simulink model "CrCtl_StM"  (R2016b)
settings: configuration reference "CodeGenConfigSet" (kept outside this file)
values from neighbouring files (symbols this model uses):
  CrCtl_aAccThres_C = Calibration.Parameter    [init_CrCtl_StM.m]
  CrCtl_aDeclThres_C = Calibration.Parameter    [init_CrCtl_StM.m]
  CrCtl_facRmpSlpAcc_C = Calibration.Parameter    [init_CrCtl_StM.m]
  CrCtl_facRmpSlpDecl_C = Calibration.Parameter    [init_CrCtl_StM.m]
  CrCtl_facRmpSlpRes_C = Calibration.Parameter    [init_CrCtl_StM.m]
  CrCtl_swtOffTipDwnTrqLim_C = Calibration.Parameter    [init_CrCtl_StM.m]
  CrCtl_swtOffTipUpTrqLim_C = Calibration.Parameter    [init_CrCtl_StM.m]
  CrCtl_trqLimOffsetAcc_C = Calibration.Parameter    [init_CrCtl_StM.m]
  CrCtl_trqLimOffsetDecl_C = Calibration.Parameter    [init_CrCtl_StM.m]
  CrCtl_vDvtMaxAccDecl_C = Calibration.Parameter    [init_CrCtl_StM.m]
  CrCtl_vMaxDvtAcc_C = Calibration.Parameter    [init_CrCtl_StM.m]
  CrCtl_vMaxDvtDecl_C = Calibration.Parameter    [init_CrCtl_StM.m]
  CrCtl_vMaxDvtResAbv_C = Calibration.Parameter    [init_CrCtl_StM.m]
  CrCtl_vMaxDvtResBlw_C = Calibration.Parameter    [init_CrCtl_StM.m]
  CrCtl_vTipDwnDvtn_C = Calibration.Parameter    [init_CrCtl_StM.m]
  CrCtl_vTipDwnLoLim_C = Calibration.Parameter    [init_CrCtl_StM.m]
  CrCtl_vTipDwnUpLim_C = Calibration.Parameter    [init_CrCtl_StM.m]
  CrCtl_vTipStp_C = Calibration.Parameter    [init_CrCtl_StM.m]
  CrCtl_vTipUpDvtn_C = Calibration.Parameter    [init_CrCtl_StM.m]
  CrCtl_vTipUpLoLim_C = Calibration.Parameter    [init_CrCtl_StM.m]
  CrCtl_vTipUpUpLim_C = Calibration.Parameter    [init_CrCtl_StM.m]
  MoFDrAs_vCCtlMinCalMsg_C = Calibration.Parameter    [init_CrCtl_StM.m]
  VEL_ZERO = fi(0,VehSpeed_km_h)    [init_CrCtl_StM.m]
undefined symbols (not defined in the file or in its folder): CrCtl_stLck_conv, CrCtl_StM_DT, CrCtl_stShOff_conv, CrCtl_stSub_conv, CruiseCtl_State_conv
libraries: CXLib x15
(part 1 of 2)
settings Model: Creator=guanxiaoxing  LastModifiedBy=guanxiaoxing
settings ConfigSetRef: SourceLocation=Base Workspace

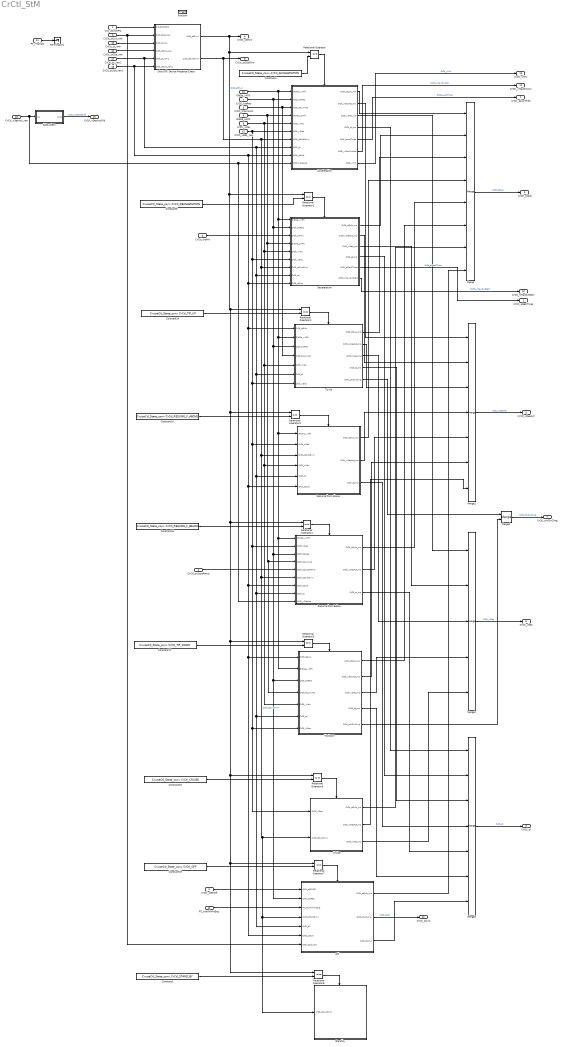
== system CrCtl_StM ==
  CrC_bCrCtlPrs : Inport  Description=Cruise control present status  OutMin=0  OutMax=1  OutDataTypeStr=boolean
  CrCtl_stLck_raw : Inport  Description=Cruise Control lock Status  Port=2  OutDataTypeStr=Enum: CrCtl_stLck_conv
  CrCtl_stShOff : Inport  Description=cruise control shut-off requirement  Port=3  OutDataTypeStr=Enum: CrCtl_stShOff_conv
  CrCtl_stSuspRamp : Inport  Description=Suspend ramp status  Port=4  OutDataTypeStr=Enum: CrCtl_stSuspRamp_conv
  CrCtl_trqLimAct : Inport  Tag=Nm  Description=Limited Cruise control torque  Port=5  OutMin=-3000  OutMax=3000  OutDataTypeStr=Trq_Nm
  CrCtl_trqMin : Inport  Tag=Nm  Description=cruise control desired torque when cruise control is inactive  Port=6  OutMin=-3000  OutMax=3000  OutDataTypeStr=Trq_Nm
  CrCtl_trqReq : Inport  Tag=Nm  Description=Cruise control torque request  Port=7  OutMin=-3000  OutMax=3000  OutDataTypeStr=Trq_Nm
  CrCtl_vMax : Inport  Tag=km/h  Description=Maximum speed for cruise control  Port=8  OutMin=0  OutMax=250  OutDataTypeStr=VehSpeed_km_h
  GlbDa_aXFlt : Inport  Tag=m/s^2  Description=Vehicle longitudinal acceleration filtered  Port=9  OutMin=-32  OutMax=32  OutDataTypeStr=Acc_m_s2
  GlbDa_vXFlt : Inport  Tag=km/h  Description=Vehicle velocity filtered  Port=10  OutMin=0  OutMax=250  OutDataTypeStr=VehSpeed_km_h
  PT_rTraV2N : Inport  Tag=km/h/rpm  Description=Quotient of velocity and engine speed  Port=11  OutMin=-0.32768  OutMax=0.32767  OutDataTypeStr=Tra_V2N_km_h_rpm
  PT_trqWhlMinEng : Inport  Tag=Nm  Description=Minimum wheel torque from the engine  Port=12  OutMin=-3000  OutMax=3000  OutDataTypeStr=Trq_Nm
  CrCtl_st_raw : Inport  Description=Application parameter for Cruise Control state  Port=13  OutDataTypeStr=Enum: CruiseCtl_State_conv
  CrCtl_stSub_raw : Inport  Description=Cruise control sub mode  Port=14  OutDataTypeStr=Enum: CrCtl_stSub_conv
  CrCtl_vDes_raw : Inport  Tag=km/h  Description=Cruise Control desired set point speed  Port=15  OutMin=0  OutMax=250  OutDataTypeStr=VehSpeed_km_h
  CrCtl_vDesAct_raw : Inport  Tag=km/h  Description=Target speed for cruise control  Port=16  OutMin=0  OutMax=250  OutDataTypeStr=VehSpeed_km_h
  CrCtl_st_raw1 : Inport  Description=Application parameter for Cruise Control state  Port=17  OutDataTypeStr=Enum: CruiseCtl_State_conv
  CrCtl_stSub_raw1 : Inport  Description=Cruise control sub mode  Port=18  OutDataTypeStr=Enum: CrCtl_stSub_conv
  function : TriggerPort  TriggerType=function-call  VariantControl=Variant
  Acceleration : Subsystem
  Constant1 : Constant  Value=CruiseCtl_State_conv.CrCtl_STAND_BY
  Constant14 : Constant  Value=CruiseCtl_State_conv.CrCtl_TIP_UP
  Constant15 : Constant  Value=CruiseCtl_State_conv.CrCtl_RESUME_F_ABOVE
  Constant16 : Constant  Value=CruiseCtl_State_conv.CrCtl_RESUME_F_BELOW
  Constant17 : Constant  Value=CruiseCtl_State_conv.CrCtl_TIP_DOWN
  Constant18 : Constant  Value=CruiseCtl_State_conv.CrCtl_CRUISE
  Constant19 : Constant  Value=CruiseCtl_State_conv.CrCtl_OFF
  Constant4 : Constant  Value=CruiseCtl_State_conv.CrCtl_ACCELERATION
  Constant6 : Constant  Value=CruiseCtl_State_conv.CrCtl_DECELERATION
  Cruise : Subsystem
  Deceleration : Subsystem
  Merge : Merge  Inputs=8
  Merge1 : Merge  Inputs=7
  Merge2 : Merge  Inputs=5
  Merge3 : Merge  Inputs=7
  Merge4 : Merge
  Off : Subsystem
  Relational Operator{,1..8} (9 alike) : RelationalOperator  Operator===  OutDataTypeStr=boolean  RndMeth=Simplest
  Resume from Above : Subsystem
  Resume from Below : Subsystem
  Shut Off / Device Presence Check : Subsystem
  Stand by : Subsystem
  Subsystem : Subsystem
  Terminator1 : Terminator
  Tip Down : Subsystem
  Tip Up : Subsystem
  CrCtl_aAccThres : Outport  Tag=m/s^2  Description=Accelration threshold for Cruise control  OutMin=-32  OutMax=32  OutDataTypeStr=Acc_m_s2
  CrCtl_aDeclThres : Outport  Tag=m/s^2  Description=Deaccelration threshold for Cruise control  Port=2  OutMin=-32  OutMax=32  OutDataTypeStr=Acc_m_s2
  CrCtl_st : Outport  Description=Application parameter for Cruise Control state  Port=3  OutDataTypeStr=Enum: CruiseCtl_State_conv
  CrCtl_stGvnr : Outport  Description=Governor status for cruise control  Port=4  OutDataTypeStr=Enum: CruiseCtl_State_conv
  CrCtl_stSub : Outport  Description=Cruise control sub mode  Port=5  OutDataTypeStr=Enum: CrCtl_stSub_conv
  CrCtl_stSubGvnr : Outport  Description=Cruise control sub mode for governor  Port=6  OutDataTypeStr=Enum: CrCtl_stSub_conv
  CrCtl_stVDirChng : Outport  Description=|  Port=7  OutMin=0  OutMax=1  OutDataTypeStr=boolean
      | Flag indicating if vehicle was under increasing speed request before and now speed decrease has
      | been request (or vice-versa)
  CrCtl_vDes : Outport  Tag=km/h  Description=Cruise Control desired set point speed  Port=8  OutMin=0  OutMax=250  OutDataTypeStr=VehSpeed_km_h
  CrCtl_vDesAct : Outport  Tag=km/h  Description=Target speed for cruise control  Port=9  OutMin=0  OutMax=250  OutDataTypeStr=VehSpeed_km_h
  CrCtl_vDesActOld : Outport  Tag=km/h  Description=Cruise control old active speed  Port=10  OutMin=0  OutMax=250  OutDataTypeStr=VehSpeed_km_h
  CrCtl_vMaxDvtAcc : Outport  Tag=km/h  Description=Maximum deviation speed for acceleration  Port=11  OutMin=0  OutMax=250  OutDataTypeStr=VehSpeed_km_h
  CrCtl_vMaxDvtDecl : Outport  Tag=km/h  Description=Maximum deviation speed for deacceleration  Port=12  OutMin=0  OutMax=250  OutDataTypeStr=VehSpeed_km_h
  CrCtl_vMin : Outport  Tag=km/h  Description=Minimum spped for cruise control  Port=13  OutMin=0  OutMax=250  OutDataTypeStr=VehSpeed_km_h
  CrCtl_stLck : Outport  Description=Cruise Control lock Status  Port=14  OutDataTypeStr=Enum: CrCtl_stLck_conv
  wires:
  Acceleration/5(CrCtl_aAccThres) -> CrCtl_aAccThres/1  "CrCtl_aAccThres"
  Deceleration/5(CrCtl_aDeclThres) -> CrCtl_aDeclThres/1  "CrCtl_aDeclThres"
  Merge3/1 -> CrCtl_st/1  "CrCtl_st"
  Shut Off / Device Presence Check/1(CrCtl_stGvnr) -> Relational Operator4/1, Relational Operator5/1, Relational Operator6/1, Relational Operator8/1, Relational Operator7/1, Relational Operator3/1, Relational Operator2/1, Relational Operator1/1, Relational Operator/1, CrCtl_stGvnr/1  "CrCtl_stGvnr"
  Merge/1 -> CrCtl_stSub/1  "CrCtl_stSub"
  Shut Off / Device Presence Check/2("CrCtl_stSubGvnr ") -> CrCtl_stSubGvnr/1, Resume from Below/6(CrCtl_stSubGvnr), Stand by/1(CrCtl_stSubGvnr), Off/4(CrCtl_stSubGvnr), Cruise/2(CrCtl_stSubGvnr), Resume from Above/3(CrCtl_stSubGvnr), Deceleration/7(CrCtl_stSubGvnr), Acceleration/7(CrCtl_stSubGvnr)  "CrCtl_stSubGvnr"
  Merge4/1 -> CrCtl_stVDirChng/1  "CrCtl_stVDirChng"
  Merge2/1 -> CrCtl_vDes/1  "CrCtl_vDes"
  Merge1/1 -> CrCtl_vDesAct/1  "CrCtl_vDesAct"
  Acceleration/6(" CrCtl_vMaxDvtAcc") -> CrCtl_vMaxDvtAcc/1  "CrCtl_vMaxDvtAcc"
  Deceleration/6(" CrCtl_vMaxDvtDecl") -> CrCtl_vMaxDvtDecl/1  "CrCtl_vMaxDvtDecl"
  Acceleration/7(" CrCtl_vMin") -> CrCtl_vMin/1  "CrCtl_vMin"
  PT_rTraV2N/1 -> Terminator1/1
  CrC_bCrCtlPrs/1 -> Shut Off / Device Presence Check/1(CrC_bCrCtlPrs)
  CrCtl_trqLimAct/1 -> Tip Up/4(CrCtl_trqLimAct), Acceleration/3(CrCtl_trqLimAct)
  GlbDa_aXFlt/1 -> Tip Down/4(CrCtl_trqLimAct), Resume from Below/4(CrCtl_trqLimAct), Deceleration/4(GlbDa_aXFlt), Acceleration/4(GlbDa_aXFlt)
  CrCtl_vMax/1 -> Tip Down/5(CrCtl_vMax), Resume from Above/4(CrCtl_vMax), Tip Up/5(CrCtl_vMax), Deceleration/5(CrCtl_vMax), Acceleration/5(CrCtl_vMax)
  CrCtl_trqMin/1 -> Deceleration/3(CrCtl_trqMin)
  CrCtl_stSuspRamp/1 -> Resume from Below/5(CrCtl_stSuspRamp)
  GlbDa_vXFlt/1 -> Resume from Below/1(GlbDa_vXFlt), Tip Down/2(GlbDa_vXFlt), Resume from Above/1(GlbDa_vXFlt), Tip Up/2(GlbDa_vXFlt), Deceleration/1(GlbDa_vXFlt), Acceleration/1(GlbDa_vXFlt)
  Constant4/1 -> Relational Operator/2
  Relational Operator/1 -> Acceleration/Enable
  CrCtl_trqReq/1 -> Off/2(CrCtl_trqReq), Tip Down/3(CrCtl_trqReq), Resume from Below/3(CrCtl_trqReq), Tip Up/3(CrCtl_trqReq), Deceleration/2(CrCtl_trqReq), Acceleration/2(CrCtl_trqReq)
  CrCtl_stShOff/1 -> Off/1(CrCtl_stShOff)
  PT_trqWhlMinEng/1 -> Off/3(PT_trqWhlMinEng)
  Constant6/1 -> Relational Operator1/2
  Relational Operator1/1 -> Deceleration/Enable
  Constant14/1 -> Relational Operator2/2
  Relational Operator2/1 -> Tip Up/Enable
  Constant15/1 -> Relational Operator3/2
  Relational Operator3/1 -> Resume from Above/Enable
  Constant16/1 -> Relational Operator4/2
  Relational Operator4/1 -> Resume from Below/Enable
  Constant17/1 -> Relational Operator5/2
  Relational Operator5/1 -> Tip Down/Enable
  Constant18/1 -> Relational Operator6/2
  Relational Operator6/1 -> Cruise/Enable
  Constant19/1 -> Relational Operator7/2
  Relational Operator7/1 -> Off/Enable
  CrCtl_stLck_raw/1 -> Off/7(CrCtl_stLck_raw), Shut Off / Device Presence Check/2(CrCtl_stLck_raw)
  Deceleration/1(CrCtl_stSub_mp) -> Merge/2
  Tip Up/1(CrCtl_stSub_mp) -> Merge/3
  Resume from Above/1(CrCtl_stSub_mp) -> Merge/4
  Resume from Below/1(CrCtl_stSub_mp) -> Merge/5
  Tip Down/1(CrCtl_stSub_mp) -> Merge/6
  Cruise/1(CrCtl_stSub_mp) -> Merge/7
  Off/1(CrCtl_stSub_mp) -> Merge/8
  Acceleration/2(CrCtl_vDesAct_mp) -> Merge1/1
  Deceleration/2(CrCtl_vDesAct_mp) -> Merge1/2
  Tip Up/2(CrCtl_vDesAct_mp) -> Merge1/3
  Resume from Above/2(CrCtl_vDesAct_mp) -> Merge1/4
  Resume from Below/2(CrCtl_vDesAct_mp) -> Merge1/5
  Tip Down/2(CrCtl_vDesAct_mp) -> Merge1/6
  Cruise/2(CrCtl_vDesAct_mp) -> Merge1/7
  Acceleration/3(CrCtl_vDes_mp) -> Merge2/1
  Deceleration/3(CrCtl_vDes_mp) -> Merge2/2
  Tip Up/3(CrCtl_vDes_mp) -> Merge2/3
  Tip Down/3(CrCtl_vDes_mp) -> Merge2/4
  Acceleration/4(CrCtl_st_mp) -> Merge3/1
  Deceleration/4(CrCtl_st_mp) -> Merge3/2
  Tip Up/4(CrCtl_st_mp) -> Merge3/3
  Resume from Above/3(CrCtl_st_mp) -> Merge3/4
  Off/3(CrCtl_st_mp) -> Merge3/7
  Resume from Below/3(CrCtl_st_mp) -> Merge3/5
  Tip Down/4(CrCtl_st_mp) -> Merge3/6
  Tip Down/5(CrCtl_stVDirChng) -> Merge4/2
  Tip Up/5(CrCtl_stVDirChng) -> Merge4/1
  CrCtl_st_raw1/1 -> Shut Off / Device Presence Check/5(CrCtl_st_raw1), Resume from Above/5(CrCtl_st), Off/5(CrCtl_st), Tip Down/6(CrCtl_st), Resume from Below/8(CrCtl_st), Tip Up/6(CrCtl_st), Deceleration/8(CrCtl_st), Acceleration/8(CrCtl_st)
  CrCtl_stSub_raw1/1 -> Shut Off / Device Presence Check/6(CrCtl_stSub_raw1), Resume from Above/6(CrCtl_stSub), Off/6(CrCtl_stSub), Tip Down/1(CrCtl_stSub), Resume from Below/7(CrCtl_stSub), Tip Up/1(CrCtl_stSub), Deceleration/9(CrCtl_stSub), Acceleration/9(CrCtl_stSub)
  Off/2(CrCtl_stLck_mp) -> CrCtl_stLck/1  "CrCtl_stLck"
  Cruise/3(CrCtl_vDes_mp) -> Merge2/5
  Constant1/1 -> Relational Operator8/2
  Relational Operator8/1 -> Stand by/Enable
  Subsystem/1(Out1) -> CrCtl_vDesActOld/1  "CrCtl_vDesActOld"
  CrCtl_vDesAct_raw/1 -> Resume from Below/9(CrCtl_vDesAct), Acceleration/10(CrCtl_vDesAct), Subsystem/1(In1)
  CrCtl_stSub_raw/1 -> Shut Off / Device Presence Check/4(CrCtl_stSub_raw)
  CrCtl_st_raw/1 -> Shut Off / Device Presence Check/3(CrCtl_st_raw)
  Acceleration/1(CrCtl_stSub_mp) -> Merge/1
  CrCtl_vDes_raw/1 -> Acceleration/6(CrCtl_vDes), Tip Up/7(CrCtl_vDes), Tip Down/7(CrCtl_vDes), Cruise/1(CrCtl_vDes), Resume from Below/2(CrCtl_vDes), Resume from Above/2(CrCtl_vDes), Deceleration/6(CrCtl_vDes)

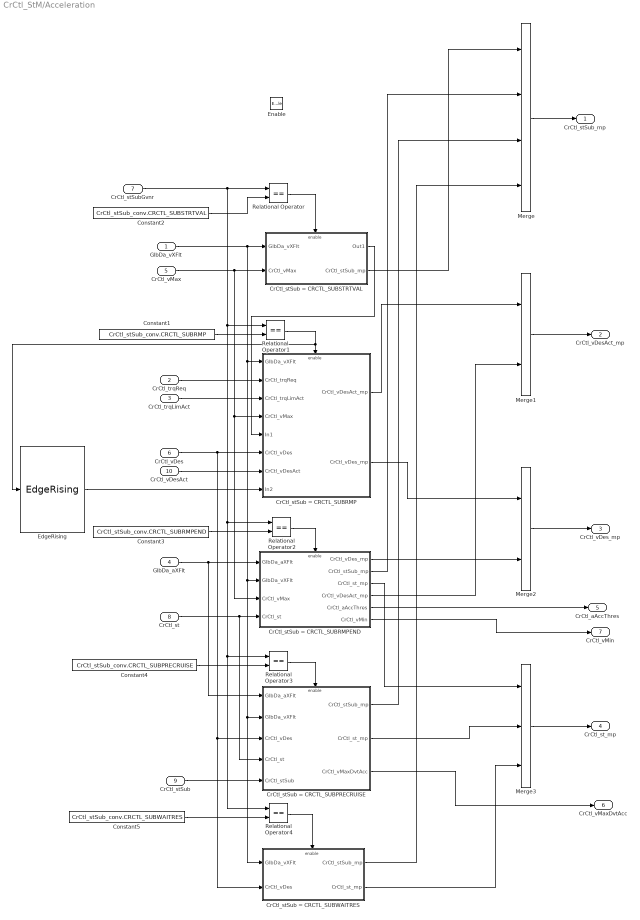
== system CrCtl_StM/Acceleration ==
  GlbDa_vXFlt : Inport
  CrCtl_trqReq : Inport  Port=2
  CrCtl_trqLimAct : Inport  Port=3
  GlbDa_aXFlt : Inport  Port=4
  CrCtl_vMax : Inport  Port=5
  CrCtl_vDes : Inport  Port=6
  CrCtl_stSubGvnr : Inport  Port=7
  CrCtl_st : Inport  Port=8
  CrCtl_stSub : Inport  Port=9
  CrCtl_vDesAct : Inport  Port=10
  Enable : EnablePort
  Constant1 : Constant  Value=CrCtl_stSub_conv.CRCTL_SUBRMP
  Constant2 : Constant  Value=CrCtl_stSub_conv.CRCTL_SUBSTRTVAL
  Constant3 : Constant  Value=CrCtl_stSub_conv.CRCTL_SUBRMPEND
  Constant4 : Constant  Value=CrCtl_stSub_conv.CRCTL_SUBPRECRUISE
  Constant5 : Constant  Value=CrCtl_stSub_conv.CRCTL_SUBWAITRES
  CrCtl_stSub = CRCTL_SUBPRECRUISE : Subsystem
  CrCtl_stSub = CRCTL_SUBRMP : Subsystem
  CrCtl_stSub = CRCTL_SUBRMPEND : Subsystem
  "CrCtl_stSub = CRCTL_SUBSTRTVAL " : Subsystem
  CrCtl_stSub = CRCTL_SUBWAITRES : Subsystem
  EdgeRising : CXLib/EdgeRising
  Merge : Merge  Inputs=4
  Merge1 : Merge
  Merge2 : Merge
  Merge3 : Merge  Inputs=3
  Relational Operator{,1..4} (5 alike) : RelationalOperator  Operator===  OutDataTypeStr=boolean  RndMeth=Simplest
  CrCtl_stSub_mp : Outport
  CrCtl_vDesAct_mp : Outport  Port=2
  CrCtl_vDes_mp : Outport  Port=3
  CrCtl_st_mp : Outport  Port=4
  CrCtl_aAccThres : Outport  Port=5  OutputWhenDisabled=reset  InitialOutput=0
  " CrCtl_vMaxDvtAcc" : Outport  Port=6
  " CrCtl_vMin" : Outport  Port=7  OutputWhenDisabled=reset  InitialOutput=0
  wires:
  GlbDa_vXFlt/1 -> CrCtl_stSub = CRCTL_SUBWAITRES/1(GlbDa_vXFlt), CrCtl_stSub = CRCTL_SUBPRECRUISE/2(GlbDa_vXFlt), CrCtl_stSub = CRCTL_SUBRMPEND/2(GlbDa_vXFlt), CrCtl_stSub = CRCTL_SUBRMP/1(GlbDa_vXFlt), "CrCtl_stSub = CRCTL_SUBSTRTVAL "/1(GlbDa_vXFlt)
  CrCtl_trqLimAct/1 -> CrCtl_stSub = CRCTL_SUBRMP/3(CrCtl_trqLimAct)
  CrCtl_trqReq/1 -> CrCtl_stSub = CRCTL_SUBRMP/2(CrCtl_trqReq)
  CrCtl_vMax/1 -> CrCtl_stSub = CRCTL_SUBRMPEND/3(CrCtl_vMax), CrCtl_stSub = CRCTL_SUBRMP/4(CrCtl_vMax), "CrCtl_stSub = CRCTL_SUBSTRTVAL "/2(CrCtl_vMax)
  GlbDa_aXFlt/1 -> CrCtl_stSub = CRCTL_SUBRMPEND/1(GlbDa_aXFlt), CrCtl_stSub = CRCTL_SUBPRECRUISE/1(GlbDa_aXFlt)
  CrCtl_vDes/1 -> CrCtl_stSub = CRCTL_SUBPRECRUISE/3(CrCtl_vDes), CrCtl_stSub = CRCTL_SUBWAITRES/2(CrCtl_vDes), CrCtl_stSub = CRCTL_SUBRMP/6(CrCtl_vDes)
  Constant2/1 -> Relational Operator/2
  Relational Operator/1 -> "CrCtl_stSub = CRCTL_SUBSTRTVAL "/Enable
  Constant1/1 -> Relational Operator1/2
  Relational Operator1/1 -> EdgeRising/1, CrCtl_stSub = CRCTL_SUBRMP/Enable
  Constant3/1 -> Relational Operator2/2
  Relational Operator2/1 -> CrCtl_stSub = CRCTL_SUBRMPEND/Enable
  Constant4/1 -> Relational Operator3/2
  Relational Operator3/1 -> CrCtl_stSub = CRCTL_SUBPRECRUISE/Enable
  CrCtl_stSubGvnr/1 -> Relational Operator4/1, Relational Operator3/1, Relational Operator2/1, Relational Operator1/1, Relational Operator/1
  Constant5/1 -> Relational Operator4/2
  Relational Operator4/1 -> CrCtl_stSub = CRCTL_SUBWAITRES/Enable
  CrCtl_st/1 -> CrCtl_stSub = CRCTL_SUBPRECRUISE/4(CrCtl_st), CrCtl_stSub = CRCTL_SUBRMPEND/4(CrCtl_st)
  CrCtl_stSub/1 -> CrCtl_stSub = CRCTL_SUBPRECRUISE/5(CrCtl_stSub)
  "CrCtl_stSub = CRCTL_SUBSTRTVAL "/2(CrCtl_stSub_mp) -> Merge/1
  CrCtl_stSub = CRCTL_SUBRMPEND/2(CrCtl_stSub_mp) -> Merge/2
  CrCtl_stSub = CRCTL_SUBPRECRUISE/1(CrCtl_stSub_mp) -> Merge/3
  CrCtl_stSub = CRCTL_SUBWAITRES/1(CrCtl_stSub_mp) -> Merge/4
  Merge/1 -> CrCtl_stSub_mp/1
  CrCtl_stSub = CRCTL_SUBRMP/1(CrCtl_vDesAct_mp) -> Merge1/1
  CrCtl_stSub = CRCTL_SUBRMPEND/4(CrCtl_vDesAct_mp) -> Merge1/2
  Merge1/1 -> CrCtl_vDesAct_mp/1
  CrCtl_stSub = CRCTL_SUBRMP/2(CrCtl_vDes_mp) -> Merge2/1
  CrCtl_stSub = CRCTL_SUBRMPEND/1(CrCtl_vDes_mp) -> Merge2/2
  Merge2/1 -> CrCtl_vDes_mp/1
  CrCtl_stSub = CRCTL_SUBRMPEND/3(CrCtl_st_mp) -> Merge3/1
  CrCtl_stSub = CRCTL_SUBPRECRUISE/2(CrCtl_st_mp) -> Merge3/2
  CrCtl_stSub = CRCTL_SUBWAITRES/2(CrCtl_st_mp) -> Merge3/3
  Merge3/1 -> CrCtl_st_mp/1
  CrCtl_stSub = CRCTL_SUBRMPEND/5(CrCtl_aAccThres) -> CrCtl_aAccThres/1
  CrCtl_stSub = CRCTL_SUBPRECRUISE/3(" CrCtl_vMaxDvtAcc") -> " CrCtl_vMaxDvtAcc"/1
  CrCtl_stSub = CRCTL_SUBRMPEND/6(" CrCtl_vMin") -> " CrCtl_vMin"/1
  CrCtl_vDesAct/1 -> CrCtl_stSub = CRCTL_SUBRMP/7(CrCtl_vDesAct)
  "CrCtl_stSub = CRCTL_SUBSTRTVAL "/1(Out1) -> CrCtl_stSub = CRCTL_SUBRMP/5(In1)
  EdgeRising/1 -> CrCtl_stSub = CRCTL_SUBRMP/8(In2)

== system CrCtl_StM/Cruise ==
  CrCtl_vDes : Inport
  CrCtl_stSubGvnr : Inport  Port=2
  Enable : EnablePort
  Constant1 : Constant  Value=CrCtl_stSub_conv.CRCTL_SUBGVNR
  Constant2 : Constant  Value=CrCtl_stSub_conv.CRCTL_SUBCALCSET
  CrCtl_stSub = CRCTL_SUBGVNR : Subsystem
  CrCtl_stSub = CRCTL_SUBSTRTVAL : Subsystem
  Relational Operator : RelationalOperator  Operator===  OutDataTypeStr=boolean  RndMeth=Simplest
  Relational Operator1 : RelationalOperator  Operator===  OutDataTypeStr=boolean  RndMeth=Simplest
  CrCtl_stSub_mp : Outport
  CrCtl_vDesAct_mp : Outport  Port=2
  CrCtl_vDes_mp : Outport  Port=3
  wires:
  Constant2/1 -> Relational Operator/2
  Relational Operator/1 -> CrCtl_stSub = CRCTL_SUBSTRTVAL/Enable
  CrCtl_stSubGvnr/1 -> Relational Operator1/1, Relational Operator/1
  Constant1/1 -> Relational Operator1/2
  Relational Operator1/1 -> CrCtl_stSub = CRCTL_SUBGVNR/Enable
  CrCtl_stSub = CRCTL_SUBSTRTVAL/1(CrCtl_vDesAct) -> CrCtl_vDesAct_mp/1
  CrCtl_stSub = CRCTL_SUBGVNR/1(CrCtl_vDes_mp) -> CrCtl_vDes_mp/1
  CrCtl_vDes/1 -> CrCtl_stSub = CRCTL_SUBGVNR/1(CrCtl_vDes), CrCtl_stSub = CRCTL_SUBSTRTVAL/1(CrCtl_vDes)
  CrCtl_stSub = CRCTL_SUBSTRTVAL/2(CrCtl_stSub_mp) -> CrCtl_stSub_mp/1

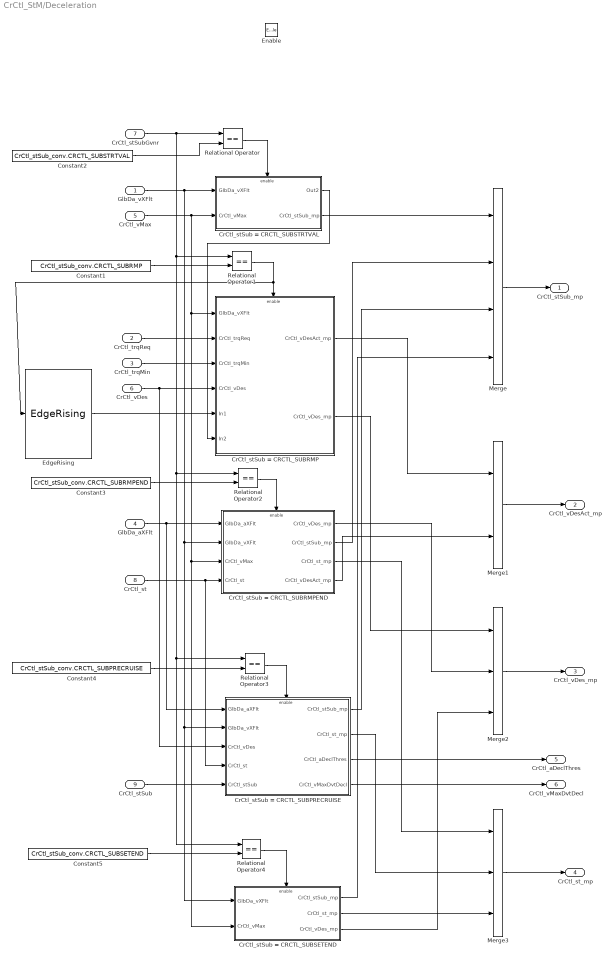
== system CrCtl_StM/Deceleration ==
  GlbDa_vXFlt : Inport
  CrCtl_trqReq : Inport  Port=2
  CrCtl_trqMin : Inport  Port=3
  GlbDa_aXFlt : Inport  Port=4
  CrCtl_vMax : Inport  Port=5
  CrCtl_vDes : Inport  Port=6
  CrCtl_stSubGvnr : Inport  Port=7
  CrCtl_st : Inport  Port=8
  CrCtl_stSub : Inport  Port=9
  Enable : EnablePort
  Constant1 : Constant  Value=CrCtl_stSub_conv.CRCTL_SUBRMP
  Constant2 : Constant  Value=CrCtl_stSub_conv.CRCTL_SUBSTRTVAL
  Constant3 : Constant  Value=CrCtl_stSub_conv.CRCTL_SUBRMPEND
  Constant4 : Constant  Value=CrCtl_stSub_conv.CRCTL_SUBPRECRUISE
  Constant5 : Constant  Value=CrCtl_stSub_conv.CRCTL_SUBSETEND
  CrCtl_stSub = CRCTL_SUBPRECRUISE : Subsystem
  CrCtl_stSub = CRCTL_SUBRMP : Subsystem
  CrCtl_stSub = CRCTL_SUBRMPEND : Subsystem
  CrCtl_stSub = CRCTL_SUBSETEND : Subsystem
  "CrCtl_stSub = CRCTL_SUBSTRTVAL " : Subsystem
  EdgeRising : CXLib/EdgeRising
  Merge : Merge  Inputs=4
  Merge1 : Merge
  Merge2 : Merge  Inputs=3
  Merge3 : Merge  Inputs=3
  Relational Operator{,1..4} (5 alike) : RelationalOperator  Operator===  OutDataTypeStr=boolean  RndMeth=Simplest
  CrCtl_stSub_mp : Outport
  CrCtl_vDesAct_mp : Outport  Port=2
  CrCtl_vDes_mp : Outport  Port=3
  CrCtl_st_mp : Outport  Port=4
  CrCtl_aDeclThres : Outport  Port=5
  " CrCtl_vMaxDvtDecl" : Outport  Port=6
  wires:
  GlbDa_vXFlt/1 -> CrCtl_stSub = CRCTL_SUBSETEND/1(GlbDa_vXFlt), CrCtl_stSub = CRCTL_SUBPRECRUISE/2(GlbDa_vXFlt), CrCtl_stSub = CRCTL_SUBRMPEND/2(GlbDa_vXFlt), "CrCtl_stSub = CRCTL_SUBSTRTVAL "/1(GlbDa_vXFlt)
  CrCtl_trqMin/1 -> CrCtl_stSub = CRCTL_SUBRMP/3(CrCtl_trqMin)
  CrCtl_trqReq/1 -> CrCtl_stSub = CRCTL_SUBRMP/2(CrCtl_trqReq)
  CrCtl_vMax/1 -> CrCtl_stSub = CRCTL_SUBRMPEND/3(CrCtl_vMax), CrCtl_stSub = CRCTL_SUBSETEND/2(CrCtl_vMax), CrCtl_stSub = CRCTL_SUBRMP/1(GlbDa_vXFlt), "CrCtl_stSub = CRCTL_SUBSTRTVAL "/2(CrCtl_vMax)
  GlbDa_aXFlt/1 -> CrCtl_stSub = CRCTL_SUBPRECRUISE/1(GlbDa_aXFlt), CrCtl_stSub = CRCTL_SUBRMPEND/1(GlbDa_aXFlt)
  CrCtl_vDes/1 -> CrCtl_stSub = CRCTL_SUBPRECRUISE/3(CrCtl_vDes), CrCtl_stSub = CRCTL_SUBRMP/4(CrCtl_vDes)
  Constant2/1 -> Relational Operator/2
  Relational Operator/1 -> "CrCtl_stSub = CRCTL_SUBSTRTVAL "/Enable
  CrCtl_st/1 -> CrCtl_stSub = CRCTL_SUBPRECRUISE/4(CrCtl_st), CrCtl_stSub = CRCTL_SUBRMPEND/4(CrCtl_st)
  CrCtl_stSub/1 -> CrCtl_stSub = CRCTL_SUBPRECRUISE/5(CrCtl_stSub)
  Constant1/1 -> Relational Operator1/2
  Constant3/1 -> Relational Operator2/2
  Relational Operator2/1 -> CrCtl_stSub = CRCTL_SUBRMPEND/Enable
  Constant4/1 -> Relational Operator3/2
  Relational Operator3/1 -> CrCtl_stSub = CRCTL_SUBPRECRUISE/Enable
  CrCtl_stSubGvnr/1 -> Relational Operator4/1, Relational Operator3/1, Relational Operator2/1, Relational Operator1/1, Relational Operator/1
  Constant5/1 -> Relational Operator4/2
  Relational Operator4/1 -> CrCtl_stSub = CRCTL_SUBSETEND/Enable
  Merge/1 -> CrCtl_stSub_mp/1
  Merge1/1 -> CrCtl_vDesAct_mp/1
  Merge2/1 -> CrCtl_vDes_mp/1
  Merge3/1 -> CrCtl_st_mp/1
  "CrCtl_stSub = CRCTL_SUBSTRTVAL "/2(CrCtl_stSub_mp) -> Merge/1
  CrCtl_stSub = CRCTL_SUBRMP/1(CrCtl_vDesAct_mp) -> Merge1/1
  CrCtl_stSub = CRCTL_SUBRMP/2(CrCtl_vDes_mp) -> Merge2/1
  CrCtl_stSub = CRCTL_SUBRMPEND/1(CrCtl_vDes_mp) -> Merge2/2
  CrCtl_stSub = CRCTL_SUBRMPEND/2(CrCtl_stSub_mp) -> Merge/2
  CrCtl_stSub = CRCTL_SUBRMPEND/3(CrCtl_st_mp) -> Merge3/1
  CrCtl_stSub = CRCTL_SUBRMPEND/4(CrCtl_vDesAct_mp) -> Merge1/2
  CrCtl_stSub = CRCTL_SUBPRECRUISE/1(CrCtl_stSub_mp) -> Merge/3
  CrCtl_stSub = CRCTL_SUBPRECRUISE/2(CrCtl_st_mp) -> Merge3/2
  CrCtl_stSub = CRCTL_SUBSETEND/2(CrCtl_st_mp) -> Merge3/3
  CrCtl_stSub = CRCTL_SUBSETEND/3(CrCtl_vDes_mp) -> Merge2/3
  CrCtl_stSub = CRCTL_SUBSETEND/1(CrCtl_stSub_mp) -> Merge/4
  CrCtl_stSub = CRCTL_SUBPRECRUISE/3(CrCtl_aDeclThres) -> CrCtl_aDeclThres/1
  CrCtl_stSub = CRCTL_SUBPRECRUISE/4(" CrCtl_vMaxDvtDecl") -> " CrCtl_vMaxDvtDecl"/1
  Relational Operator1/1 -> EdgeRising/1, CrCtl_stSub = CRCTL_SUBRMP/Enable
  EdgeRising/1 -> CrCtl_stSub = CRCTL_SUBRMP/5(In1)
  "CrCtl_stSub = CRCTL_SUBSTRTVAL "/1(Out2) -> CrCtl_stSub = CRCTL_SUBRMP/6(In2)

== system CrCtl_StM/Off ==
  CrCtl_stShOff : Inport
  CrCtl_trqReq : Inport  Port=2
  PT_trqWhlMinEng : Inport  Port=3
  CrCtl_stSubGvnr : Inport  Port=4
  CrCtl_st : Inport  Port=5
  CrCtl_stSub : Inport  Port=6
  CrCtl_stLck_raw : Inport  Port=7
  Enable : EnablePort
  Constant1 : Constant  Value=CrCtl_stSub_conv.CRCTL_SUBRMP
  Constant2 : Constant  Value=CrCtl_stSub_conv.CRCTL_SUBSTRTVAL
  CrCtl_stSub = CRCTL_SUBRMP : Subsystem
  CrCtl_stSub = CRCTL_SUBSTRTVAL : Subsystem
  Merge : Merge
  Merge1 : Merge
  Relational Operator : RelationalOperator  Operator===  OutDataTypeStr=boolean  RndMeth=Simplest
  Relational Operator1 : RelationalOperator  Operator===  OutDataTypeStr=boolean  RndMeth=Simplest
  CrCtl_stSub_mp : Outport
  CrCtl_stLck_mp : Outport  Port=2
  CrCtl_st_mp : Outport  Port=3
  wires:
  CrCtl_stShOff/1 -> CrCtl_stSub = CRCTL_SUBSTRTVAL/1("CrCtl_stShOff ")
  Constant2/1 -> Relational Operator/2
  Relational Operator/1 -> CrCtl_stSub = CRCTL_SUBSTRTVAL/Enable
  CrCtl_stSubGvnr/1 -> Relational Operator/1, Relational Operator1/1
  Constant1/1 -> Relational Operator1/2
  Relational Operator1/1 -> CrCtl_stSub = CRCTL_SUBRMP/Enable
  CrCtl_trqReq/1 -> CrCtl_stSub = CRCTL_SUBRMP/1(CrCtl_trqReq)
  PT_trqWhlMinEng/1 -> CrCtl_stSub = CRCTL_SUBRMP/2(PT_trqWhlMinEng)
  CrCtl_stLck_raw/1 -> CrCtl_stSub = CRCTL_SUBSTRTVAL/4(CrCtl_stLck_raw)
  CrCtl_st/1 -> CrCtl_stSub = CRCTL_SUBSTRTVAL/2(CrCtl_st)
  CrCtl_stSub/1 -> CrCtl_stSub = CRCTL_SUBSTRTVAL/3(CrCtl_stSub)
  Merge/1 -> CrCtl_stSub_mp/1
  CrCtl_stSub = CRCTL_SUBSTRTVAL/3(CrCtl_stLck_mp) -> CrCtl_stLck_mp/1
  CrCtl_stSub = CRCTL_SUBSTRTVAL/1(CrCtl_stSub_mp) -> Merge/1
  CrCtl_stSub = CRCTL_SUBRMP/1(CrCtl_stSub_mp) -> Merge/2
  CrCtl_stSub = CRCTL_SUBRMP/2(CrCtl_st_mp) -> Merge1/2
  CrCtl_stSub = CRCTL_SUBSTRTVAL/2(CrCtl_st_mp) -> Merge1/1
  Merge1/1 -> CrCtl_st_mp/1

== system CrCtl_StM/Resume from Above ==
  GlbDa_vXFlt : Inport
  CrCtl_vDes : Inport  Port=2
  CrCtl_stSubGvnr : Inport  Port=3
  CrCtl_vMax : Inport  Port=4
  CrCtl_st : Inport  Port=5
  CrCtl_stSub : Inport  Port=6
  Enable : EnablePort
  Constant1 : Constant  Value=CrCtl_stSub_conv.CRCTL_SUBRMP
  Constant2 : Constant  Value=CrCtl_stSub_conv.CRCTL_SUBSTRTVAL
  CrCtl_stSub = CRCTL_SUBRMP : Subsystem
  CrCtl_stSub = CRCTL_SUBSTRTVAL : Subsystem
  EdgeRising : CXLib/EdgeRising
  Merge : Merge
  Relational Operator : RelationalOperator  Operator===  OutDataTypeStr=boolean  RndMeth=Simplest
  Relational Operator1 : RelationalOperator  Operator===  OutDataTypeStr=boolean  RndMeth=Simplest
  CrCtl_stSub_mp : Outport
  CrCtl_vDesAct_mp : Outport  Port=2
  CrCtl_st_mp : Outport  Port=3
  wires:
  GlbDa_vXFlt/1 -> CrCtl_stSub = CRCTL_SUBSTRTVAL/1(GlbDa_vXFlt), CrCtl_stSub = CRCTL_SUBRMP/1(GlbDa_vXFlt)
  CrCtl_vDes/1 -> CrCtl_stSub = CRCTL_SUBRMP/2(CrCtl_vDes), CrCtl_stSub = CRCTL_SUBSTRTVAL/2(CrCtl_vDes)
  Constant2/1 -> Relational Operator/2
  CrCtl_stSubGvnr/1 -> Relational Operator1/1, Relational Operator/1
  Constant1/1 -> Relational Operator1/2
  Relational Operator1/1 -> EdgeRising/1, CrCtl_stSub = CRCTL_SUBRMP/Enable
  Relational Operator/1 -> CrCtl_stSub = CRCTL_SUBSTRTVAL/Enable
  CrCtl_vMax/1 -> CrCtl_stSub = CRCTL_SUBSTRTVAL/3(CrCtl_vMax)
  CrCtl_stSub = CRCTL_SUBSTRTVAL/2(CrCtl_vDesAct) -> CrCtl_stSub = CRCTL_SUBRMP/3(In)
  CrCtl_stSub = CRCTL_SUBRMP/1(CrCtl_vDesAct_mp) -> CrCtl_vDesAct_mp/1
  CrCtl_stSub = CRCTL_SUBRMP/2(CrCtl_st_mp) -> CrCtl_st_mp/1
  CrCtl_stSub = CRCTL_SUBRMP/3(CrCtl_stSub_mp) -> Merge/2
  CrCtl_stSub = CRCTL_SUBSTRTVAL/1(CrCtl_stSub_mp) -> Merge/1
  Merge/1 -> CrCtl_stSub_mp/1
  CrCtl_st/1 -> CrCtl_stSub = CRCTL_SUBRMP/4(CrCtl_st)
  CrCtl_stSub/1 -> CrCtl_stSub = CRCTL_SUBRMP/5(CrCtl_stSub)
  EdgeRising/1 -> CrCtl_stSub = CRCTL_SUBRMP/6(In1)

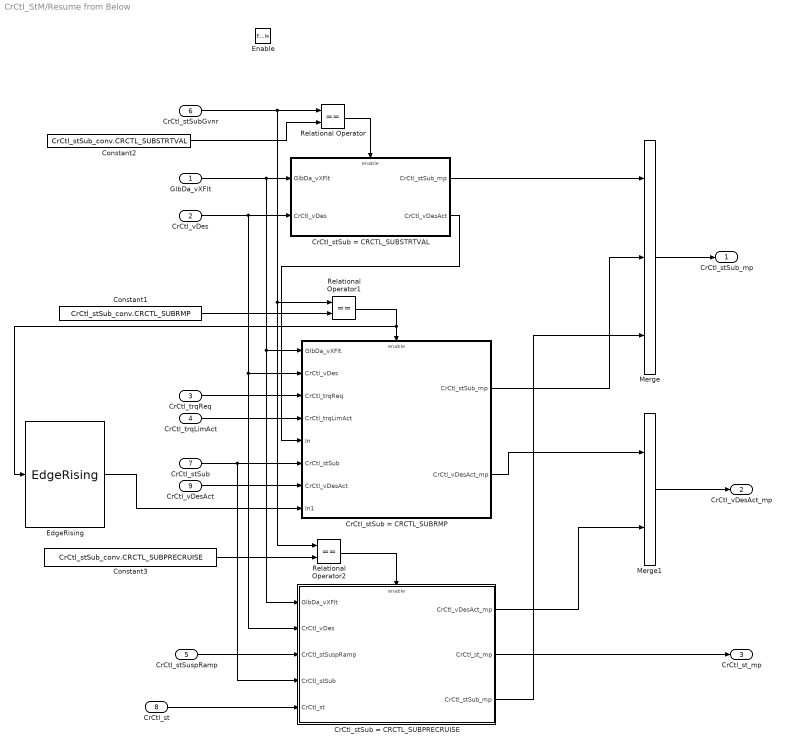
== system CrCtl_StM/Resume from Below ==
  GlbDa_vXFlt : Inport
  CrCtl_vDes : Inport  Port=2
  CrCtl_trqReq : Inport  Port=3
  CrCtl_trqLimAct : Inport  Port=4
  CrCtl_stSuspRamp : Inport  Port=5
  CrCtl_stSubGvnr : Inport  Port=6
  CrCtl_stSub : Inport  Port=7
  CrCtl_st : Inport  Port=8
  CrCtl_vDesAct : Inport  Port=9
  Enable : EnablePort
  Constant1 : Constant  Value=CrCtl_stSub_conv.CRCTL_SUBRMP
  Constant2 : Constant  Value=CrCtl_stSub_conv.CRCTL_SUBSTRTVAL
  Constant3 : Constant  Value=CrCtl_stSub_conv.CRCTL_SUBPRECRUISE
  CrCtl_stSub = CRCTL_SUBPRECRUISE : Subsystem
  CrCtl_stSub = CRCTL_SUBRMP : Subsystem
  CrCtl_stSub = CRCTL_SUBSTRTVAL : Subsystem
  EdgeRising : CXLib/EdgeRising
  Merge : Merge  Inputs=3
  Merge1 : Merge
  Relational Operator : RelationalOperator  Operator===  OutDataTypeStr=boolean  RndMeth=Simplest
  Relational Operator1 : RelationalOperator  Operator===  OutDataTypeStr=boolean  RndMeth=Simplest
  Relational Operator2 : RelationalOperator  Operator===  OutDataTypeStr=boolean  RndMeth=Simplest
  CrCtl_stSub_mp : Outport
  CrCtl_vDesAct_mp : Outport  Port=2
  CrCtl_st_mp : Outport  Port=3
  wires:
  GlbDa_vXFlt/1 -> CrCtl_stSub = CRCTL_SUBPRECRUISE/1(GlbDa_vXFlt), CrCtl_stSub = CRCTL_SUBRMP/1(GlbDa_vXFlt), CrCtl_stSub = CRCTL_SUBSTRTVAL/1(GlbDa_vXFlt)
  CrCtl_vDes/1 -> CrCtl_stSub = CRCTL_SUBPRECRUISE/2(CrCtl_vDes), CrCtl_stSub = CRCTL_SUBRMP/2(CrCtl_vDes), CrCtl_stSub = CRCTL_SUBSTRTVAL/2(CrCtl_vDes)
  CrCtl_trqLimAct/1 -> CrCtl_stSub = CRCTL_SUBRMP/4(CrCtl_trqLimAct)
  CrCtl_trqReq/1 -> CrCtl_stSub = CRCTL_SUBRMP/3(CrCtl_trqReq)
  CrCtl_stSuspRamp/1 -> CrCtl_stSub = CRCTL_SUBPRECRUISE/3(CrCtl_stSuspRamp)
  Constant2/1 -> Relational Operator/2
  Relational Operator/1 -> CrCtl_stSub = CRCTL_SUBSTRTVAL/Enable
  Constant1/1 -> Relational Operator1/2
  Relational Operator1/1 -> EdgeRising/1, CrCtl_stSub = CRCTL_SUBRMP/Enable
  CrCtl_stSubGvnr/1 -> Relational Operator2/1, Relational Operator1/1, Relational Operator/1
  Constant3/1 -> Relational Operator2/2
  Relational Operator2/1 -> CrCtl_stSub = CRCTL_SUBPRECRUISE/Enable
  CrCtl_stSub = CRCTL_SUBSTRTVAL/2(CrCtl_vDesAct) -> CrCtl_stSub = CRCTL_SUBRMP/5(In)
  CrCtl_stSub/1 -> CrCtl_stSub = CRCTL_SUBPRECRUISE/4(CrCtl_stSub), CrCtl_stSub = CRCTL_SUBRMP/6(CrCtl_stSub)
  CrCtl_st/1 -> CrCtl_stSub = CRCTL_SUBPRECRUISE/5(CrCtl_st)
  Merge/1 -> CrCtl_stSub_mp/1
  Merge1/1 -> CrCtl_vDesAct_mp/1
  CrCtl_stSub = CRCTL_SUBPRECRUISE/2(CrCtl_st_mp) -> CrCtl_st_mp/1
  CrCtl_stSub = CRCTL_SUBSTRTVAL/1(CrCtl_stSub_mp) -> Merge/1
  CrCtl_stSub = CRCTL_SUBRMP/1(CrCtl_stSub_mp) -> Merge/2
  CrCtl_stSub = CRCTL_SUBRMP/2(CrCtl_vDesAct_mp) -> Merge1/1
  CrCtl_stSub = CRCTL_SUBPRECRUISE/1(CrCtl_vDesAct_mp) -> Merge1/2
  CrCtl_stSub = CRCTL_SUBPRECRUISE/3(CrCtl_stSub_mp) -> Merge/3
  CrCtl_vDesAct/1 -> CrCtl_stSub = CRCTL_SUBRMP/7(CrCtl_vDesAct)
  EdgeRising/1 -> CrCtl_stSub = CRCTL_SUBRMP/8(In1)

== system CrCtl_StM/Shut Off // Device Presence Check ==
  CrC_bCrCtlPrs : Inport
  CrCtl_stLck_raw : Inport  Port=2
  CrCtl_st_raw : Inport  Port=3
  CrCtl_stSub_raw : Inport  Port=4
  CrCtl_st_raw1 : Inport  Port=5
  CrCtl_stSub_raw1 : Inport  Port=6
  Constant : Constant  Value=CrCtl_stLck_conv.CRCTL_LCK
  Constant1 : Constant  Value=CruiseCtl_State_conv.CrCtl_STAND_BY
  Constant2 : Constant  Value=CrCtl_stSub_conv.CRCTL_SUBNOSUB
  Logical Operator : Logic  Operator=OR  AllPortsSameDT=off  OutDataTypeStr=boolean
  Logical Operator1 : Logic  Operator=NOT  AllPortsSameDT=off  OutDataTypeStr=boolean
  Relational Operator : RelationalOperator  Operator===  OutDataTypeStr=boolean  RndMeth=Simplest
  Switch : Switch  Criteria=u2 ~= 0
  Switch1 : Switch  Criteria=u2 ~= 0
  Terminator : Terminator
  Terminator1 : Terminator
  CrCtl_stGvnr : Outport
  "CrCtl_stSubGvnr " : Outport  Port=2
  wires:
  CrC_bCrCtlPrs/1 -> Logical Operator1/1
  CrCtl_stLck_raw/1 -> Relational Operator/1
  Constant/1 -> Relational Operator/2
  Relational Operator/1 -> Logical Operator/2
  Logical Operator/1 -> Switch1/2, Switch/2
  Logical Operator1/1 -> Logical Operator/1
  Constant1/1 -> Switch/1
  Switch/1 -> CrCtl_stGvnr/1
  Constant2/1 -> Switch1/1
  Switch1/1 -> "CrCtl_stSubGvnr "/1
  CrCtl_st_raw1/1 -> Switch/3
  CrCtl_st_raw/1 -> Terminator/1
  CrCtl_stSub_raw1/1 -> Switch1/3
  CrCtl_stSub_raw/1 -> Terminator1/1

== system CrCtl_StM/Stand by ==
  CrCtl_stSubGvnr : Inport
  Enable : EnablePort
  CRCTL_SUBNOSUB : Subsystem
  Constant2 : Constant  Value=CrCtl_stSub_conv.CRCTL_SUBNOSUB
  Relational Operator : RelationalOperator  Operator===  OutDataTypeStr=boolean  RndMeth=Simplest
  wires:
  CrCtl_stSubGvnr/1 -> Relational Operator/1
  Constant2/1 -> Relational Operator/2
  Relational Operator/1 -> CRCTL_SUBNOSUB/Enable

== system CrCtl_StM/Subsystem ==
  In1 : Inport
  Signal Conversion : SignalConversion  OverrideOpt=off
  Out1 : Outport
  wires:
  In1/1 -> Signal Conversion/1
  Signal Conversion/1 -> Out1/1

== system CrCtl_StM/Tip Down ==
  CrCtl_stSub : Inport
  GlbDa_vXFlt : Inport  Port=2
  CrCtl_trqReq : Inport  Port=3
  CrCtl_trqLimAct : Inport  Port=4
  CrCtl_vMax : Inport  Port=5
  CrCtl_st : Inport  Port=6
  CrCtl_vDes : Inport  Port=7
  Enable : EnablePort
  CrCtl_stSub = CRCTL_SUBCALCSET : Subsystem
  CrCtl_stSub_mp : Outport
  CrCtl_vDesAct_mp : Outport  Port=2
  CrCtl_vDes_mp : Outport  Port=3
  CrCtl_st_mp : Outport  Port=4
  CrCtl_stVDirChng : Outport  Port=5
  wires:
  CrCtl_stSub/1 -> CrCtl_stSub = CRCTL_SUBCALCSET/1(CrCtl_stSub)
  GlbDa_vXFlt/1 -> CrCtl_stSub = CRCTL_SUBCALCSET/2(GlbDa_vXFlt)
  CrCtl_trqReq/1 -> CrCtl_stSub = CRCTL_SUBCALCSET/3(CrCtl_trqReq)
  CrCtl_trqLimAct/1 -> CrCtl_stSub = CRCTL_SUBCALCSET/4(CrCtl_trqLimAct)
  CrCtl_vMax/1 -> CrCtl_stSub = CRCTL_SUBCALCSET/5(CrCtl_vMax)
  CrCtl_st/1 -> CrCtl_stSub = CRCTL_SUBCALCSET/6(CrCtl_st)
  CrCtl_stSub = CRCTL_SUBCALCSET/1(CrCtl_stSub_mp) -> CrCtl_stSub_mp/1
  CrCtl_stSub = CRCTL_SUBCALCSET/3(CrCtl_vDesAct_mp) -> CrCtl_vDesAct_mp/1
  CrCtl_stSub = CRCTL_SUBCALCSET/4(CrCtl_vDes_mp) -> CrCtl_vDes_mp/1
  CrCtl_stSub = CRCTL_SUBCALCSET/2(CrCtl_st_mp) -> CrCtl_st_mp/1
  CrCtl_stSub = CRCTL_SUBCALCSET/5(CrCtl_stVDirChng) -> CrCtl_stVDirChng/1
  CrCtl_vDes/1 -> CrCtl_stSub = CRCTL_SUBCALCSET/7(CrCtl_vDes)

== system CrCtl_StM/Tip Up ==
  CrCtl_stSub : Inport
  GlbDa_vXFlt : Inport  Port=2
  CrCtl_trqReq : Inport  Port=3
  CrCtl_trqLimAct : Inport  Port=4
  CrCtl_vMax : Inport  Port=5
  CrCtl_st : Inport  Port=6
  CrCtl_vDes : Inport  Port=7
  Enable : EnablePort
  CrCtl_stSub = CRCTL_SUBCALCSET : Subsystem
  CrCtl_stSub_mp : Outport
  CrCtl_vDesAct_mp : Outport  Port=2
  CrCtl_vDes_mp : Outport  Port=3
  CrCtl_st_mp : Outport  Port=4
  CrCtl_stVDirChng : Outport  Port=5
  wires:
  CrCtl_stSub/1 -> CrCtl_stSub = CRCTL_SUBCALCSET/1(CrCtl_stSub)
  GlbDa_vXFlt/1 -> CrCtl_stSub = CRCTL_SUBCALCSET/2(GlbDa_vXFlt)
  CrCtl_trqReq/1 -> CrCtl_stSub = CRCTL_SUBCALCSET/3(CrCtl_trqReq)
  CrCtl_trqLimAct/1 -> CrCtl_stSub = CRCTL_SUBCALCSET/4(CrCtl_trqLimAct)
  CrCtl_vMax/1 -> CrCtl_stSub = CRCTL_SUBCALCSET/5(CrCtl_vMax)
  CrCtl_st/1 -> CrCtl_stSub = CRCTL_SUBCALCSET/6(CrCtl_st)
  CrCtl_stSub = CRCTL_SUBCALCSET/1(CrCtl_stSub_mp) -> CrCtl_stSub_mp/1
  CrCtl_stSub = CRCTL_SUBCALCSET/3(CrCtl_vDesAct_mp) -> CrCtl_vDesAct_mp/1
  CrCtl_stSub = CRCTL_SUBCALCSET/4(CrCtl_vDes_mp) -> CrCtl_vDes_mp/1
  CrCtl_stSub = CRCTL_SUBCALCSET/2(CrCtl_st_mp) -> CrCtl_st_mp/1
  CrCtl_stSub = CRCTL_SUBCALCSET/5(CrCtl_stVDirChng) -> CrCtl_stVDirChng/1
  CrCtl_vDes/1 -> CrCtl_stSub = CRCTL_SUBCALCSET/7(CrCtl_vDes)

== system CrCtl_StM/Acceleration/CrCtl_stSub = CRCTL_SUBPRECRUISE ==
  GlbDa_aXFlt : Inport
  GlbDa_vXFlt : Inport  Port=2
  CrCtl_vDes : Inport  Port=3
  CrCtl_st : Inport  Port=4
  CrCtl_stSub : Inport  Port=5
  Enable : EnablePort
  Add : Sum
  Constant1 : Constant  Value=CrCtl_aAccThres_C
  Constant2 : Constant  Value=CrCtl_vMaxDvtAcc_C
  Constant4 : Constant  Value=CruiseCtl_State_conv.CrCtl_CRUISE
  Constant5 : Constant  Value=CrCtl_stSub_conv.CRCTL_SUBSTRTVAL
  Logical Operator : Logic  AllPortsSameDT=off  OutDataTypeStr=boolean
  Relational Operator : RelationalOperator  Operator=<=  OutDataTypeStr=boolean  RndMeth=Simplest
  Relational Operator1 : RelationalOperator  Operator=<=  OutDataTypeStr=boolean  RndMeth=Simplest
  Switch : Switch  Criteria=u2 ~= 0
  Switch1 : Switch  Criteria=u2 ~= 0
  CrCtl_stSub_mp : Outport
  CrCtl_st_mp : Outport  Port=2
  " CrCtl_vMaxDvtAcc" : Outport  Port=3  OutputWhenDisabled=reset  InitialOutput=0
  wires:
  GlbDa_aXFlt/1 -> Relational Operator/1
  Constant1/1 -> Relational Operator/2
  GlbDa_vXFlt/1 -> Relational Operator1/1
  Add/1 -> Relational Operator1/2
  CrCtl_vDes/1 -> Add/1
  Constant2/1 -> Add/2, " CrCtl_vMaxDvtAcc"/1
  Relational Operator1/1 -> Logical Operator/1
  Relational Operator/1 -> Logical Operator/2
  Logical Operator/1 -> Switch1/2, Switch/2
  Constant5/1 -> Switch/1
  CrCtl_stSub/1 -> Switch/3
  Switch/1 -> CrCtl_stSub_mp/1
  CrCtl_st/1 -> Switch1/3
  Constant4/1 -> Switch1/1
  Switch1/1 -> CrCtl_st_mp/1

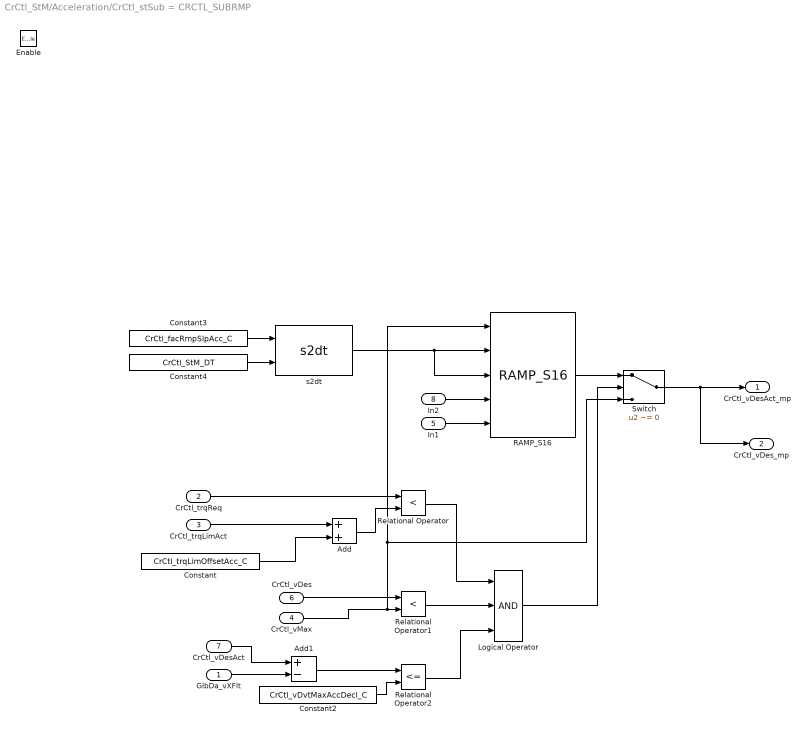
== system CrCtl_StM/Acceleration/CrCtl_stSub = CRCTL_SUBRMP ==
  GlbDa_vXFlt : Inport
  CrCtl_trqReq : Inport  Port=2
  CrCtl_trqLimAct : Inport  Port=3
  CrCtl_vMax : Inport  Port=4
  In1 : Inport  Port=5
  CrCtl_vDes : Inport  Port=6
  CrCtl_vDesAct : Inport  Port=7
  In2 : Inport  Port=8
  Enable : EnablePort
  Add : Sum
  Add1 : Sum  Inputs=+-
  Constant : Constant  Value=CrCtl_trqLimOffsetAcc_C
  Constant2 : Constant  Value=CrCtl_vDvtMaxAccDecl_C
  Constant3 : Constant  Value=CrCtl_facRmpSlpAcc_C
  Constant4 : Constant  Value=CrCtl_StM_DT
  Logical Operator : Logic  Inputs=3  AllPortsSameDT=off  OutDataTypeStr=boolean
  RAMP_S16 : CXLib/RAMP_S16
  Relational Operator : RelationalOperator  Operator=<  OutDataTypeStr=boolean  RndMeth=Simplest
  Relational Operator1 : RelationalOperator  Operator=<  OutDataTypeStr=boolean  RndMeth=Simplest
  Relational Operator2 : RelationalOperator  Operator=<=  OutDataTypeStr=boolean  RndMeth=Simplest
  Switch : Switch  Criteria=u2 ~= 0
  s2dt : CXLib/s2dt
  CrCtl_vDesAct_mp : Outport
  CrCtl_vDes_mp : Outport  Port=2
  wires:
  CrCtl_trqReq/1 -> Relational Operator/1
  CrCtl_trqLimAct/1 -> Add/1
  Constant/1 -> Add/2
  Add/1 -> Relational Operator/2
  Relational Operator/1 -> Logical Operator/1
  Relational Operator1/1 -> Logical Operator/2
  CrCtl_vMax/1 -> RAMP_S16/1, Switch/3, Relational Operator1/2
  Add1/1 -> Relational Operator2/1
  Constant2/1 -> Relational Operator2/2
  Relational Operator2/1 -> Logical Operator/3
  s2dt/1 -> RAMP_S16/3, RAMP_S16/2
  Constant3/1 -> s2dt/1
  Constant4/1 -> s2dt/2
  Logical Operator/1 -> Switch/2
  GlbDa_vXFlt/1 -> Add1/2
  In1/1 -> RAMP_S16/5
  Switch/1 -> CrCtl_vDesAct_mp/1, CrCtl_vDes_mp/1
  CrCtl_vDesAct/1 -> Add1/1
  CrCtl_vDes/1 -> Relational Operator1/1
  RAMP_S16/1 -> Switch/1
  In2/1 -> RAMP_S16/4

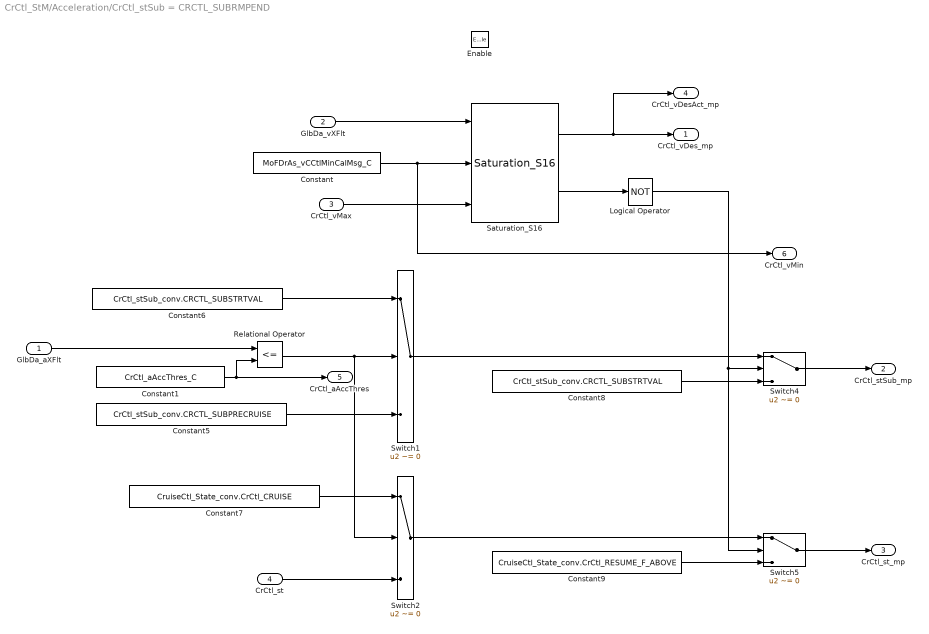
== system CrCtl_StM/Acceleration/CrCtl_stSub = CRCTL_SUBRMPEND ==
  GlbDa_aXFlt : Inport
  GlbDa_vXFlt : Inport  Port=2
  CrCtl_vMax : Inport  Port=3
  CrCtl_st : Inport  Port=4
  Enable : EnablePort
  Constant : Constant  Value=MoFDrAs_vCCtlMinCalMsg_C
  Constant1 : Constant  Value=CrCtl_aAccThres_C
  Constant5 : Constant  Value=CrCtl_stSub_conv.CRCTL_SUBPRECRUISE
  Constant6 : Constant  Value=CrCtl_stSub_conv.CRCTL_SUBSTRTVAL
  Constant7 : Constant  Value=CruiseCtl_State_conv.CrCtl_CRUISE
  Constant8 : Constant  Value=CrCtl_stSub_conv.CRCTL_SUBSTRTVAL
  Constant9 : Constant  Value=CruiseCtl_State_conv.CrCtl_RESUME_F_ABOVE
  Logical Operator : Logic  Operator=NOT  AllPortsSameDT=off  OutDataTypeStr=boolean
  Relational Operator : RelationalOperator  Operator=<=  OutDataTypeStr=boolean  RndMeth=Simplest
  Saturation_S16 : CXLib/Saturation_S16
  Switch{1..2,4..5} (4 alike) : Switch  Criteria=u2 ~= 0
  CrCtl_vDes_mp : Outport
  CrCtl_stSub_mp : Outport  Port=2
  CrCtl_st_mp : Outport  Port=3
  CrCtl_vDesAct_mp : Outport  Port=4
  CrCtl_aAccThres : Outport  Port=5  OutputWhenDisabled=reset  InitialOutput=0
  " CrCtl_vMin" : Outport  Port=6  OutputWhenDisabled=reset  InitialOutput=0
  wires:
  GlbDa_vXFlt/1 -> Saturation_S16/1
  CrCtl_vMax/1 -> Saturation_S16/3
  Saturation_S16/1 -> CrCtl_vDesAct_mp/1, CrCtl_vDes_mp/1
  Saturation_S16/2 -> Logical Operator/1
  GlbDa_aXFlt/1 -> Relational Operator/1
  Relational Operator/1 -> Switch2/2, Switch1/2
  Constant5/1 -> Switch1/3
  Constant6/1 -> Switch1/1
  Constant7/1 -> Switch2/1
  Switch1/1 -> Switch4/1
  Constant8/1 -> Switch4/3
  Logical Operator/1 -> Switch5/2, Switch4/2
  Constant9/1 -> Switch5/3
  Switch2/1 -> Switch5/1
  Switch4/1 -> CrCtl_stSub_mp/1
  Switch5/1 -> CrCtl_st_mp/1
  CrCtl_st/1 -> Switch2/3
  Constant1/1 -> CrCtl_aAccThres/1, Relational Operator/2
  Constant/1 -> " CrCtl_vMin"/1, Saturation_S16/2

== system CrCtl_StM/Acceleration/CrCtl_stSub = CRCTL_SUBSTRTVAL  ==
  GlbDa_vXFlt : Inport
  CrCtl_vMax : Inport  Port=2
  Enable : EnablePort
  Constant1 : Constant  Value=CrCtl_stSub_conv.CRCTL_SUBRMP
  MinMax : MinMax  Inputs=2
  Out1 : Outport
  CrCtl_stSub_mp : Outport  Port=2  InitialOutput=0
  wires:
  GlbDa_vXFlt/1 -> MinMax/1
  CrCtl_vMax/1 -> MinMax/2
  MinMax/1 -> Out1/1
  Constant1/1 -> CrCtl_stSub_mp/1

== system CrCtl_StM/Acceleration/CrCtl_stSub = CRCTL_SUBWAITRES ==
  GlbDa_vXFlt : Inport
  CrCtl_vDes : Inport  Port=2
  Enable : EnablePort
  Constant1 : Constant  Value=CruiseCtl_State_conv.CrCtl_RESUME_F_BELOW
  Constant3 : Constant  Value=CrCtl_stSub_conv.CRCTL_SUBPRECRUISE
  Constant4 : Constant  Value=CruiseCtl_State_conv.CrCtl_RESUME_F_ABOVE
  Relational Operator1 : RelationalOperator  Operator=>  OutDataTypeStr=boolean  RndMeth=Simplest
  Switch : Switch  Criteria=u2 ~= 0
  CrCtl_stSub_mp : Outport
  CrCtl_st_mp : Outport  Port=2
  wires:
  GlbDa_vXFlt/1 -> Relational Operator1/1
  CrCtl_vDes/1 -> Relational Operator1/2
  Relational Operator1/1 -> Switch/2
  Constant4/1 -> Switch/3
  Constant1/1 -> Switch/1
  Switch/1 -> CrCtl_st_mp/1
  Constant3/1 -> CrCtl_stSub_mp/1

== system CrCtl_StM/Cruise/CrCtl_stSub = CRCTL_SUBGVNR ==
  CrCtl_vDes : Inport
  Enable : EnablePort
  CrCtl_vDes_mp : Outport
  wires:
  CrCtl_vDes/1 -> CrCtl_vDes_mp/1

== system CrCtl_StM/Cruise/CrCtl_stSub = CRCTL_SUBSTRTVAL ==
  CrCtl_vDes : Inport
  Enable : EnablePort
  Constant3 : Constant  Value=CrCtl_stSub_conv.CRCTL_SUBSTRTVAL
  CrCtl_vDesAct : Outport
  CrCtl_stSub_mp : Outport  Port=2
  wires:
  CrCtl_vDes/1 -> CrCtl_vDesAct/1
  Constant3/1 -> CrCtl_stSub_mp/1

== system CrCtl_StM/Deceleration/CrCtl_stSub = CRCTL_SUBPRECRUISE ==
  GlbDa_aXFlt : Inport
  GlbDa_vXFlt : Inport  Port=2
  CrCtl_vDes : Inport  Port=3
  CrCtl_st : Inport  Port=4
  CrCtl_stSub : Inport  Port=5
  Enable : EnablePort
  Add : Sum  Inputs=+-
  Constant1 : Constant  Value=CrCtl_aDeclThres_C
  Constant2 : Constant  Value=CrCtl_vMaxDvtDecl_C
  Constant3 : Constant  Value=CrCtl_stSub_conv.CRCTL_SUBPRECRUISE
  Constant4 : Constant  Value=CruiseCtl_State_conv.CrCtl_CRUISE
  Logical Operator : Logic  AllPortsSameDT=off  OutDataTypeStr=boolean
  Relational Operator : RelationalOperator  OutDataTypeStr=boolean  RndMeth=Simplest
  Relational Operator1 : RelationalOperator  Operator=>  OutDataTypeStr=boolean  RndMeth=Simplest
  Switch : Switch  Criteria=u2 ~= 0
  Switch1 : Switch  Criteria=u2 ~= 0
  CrCtl_stSub_mp : Outport
  CrCtl_st_mp : Outport  Port=2
  CrCtl_aDeclThres : Outport  Port=3
  " CrCtl_vMaxDvtDecl" : Outport  Port=4
  wires:
  GlbDa_aXFlt/1 -> Relational Operator/1
  Constant1/1 -> CrCtl_aDeclThres/1, Relational Operator/2
  GlbDa_vXFlt/1 -> Relational Operator1/1
  Add/1 -> Relational Operator1/2
  CrCtl_vDes/1 -> Add/1
  Constant2/1 -> " CrCtl_vMaxDvtDecl"/1, Add/2
  Relational Operator1/1 -> Logical Operator/1
  Relational Operator/1 -> Logical Operator/2
  Logical Operator/1 -> Switch1/2, Switch/2
  Constant3/1 -> Switch/1
  Switch/1 -> CrCtl_stSub_mp/1
  CrCtl_st/1 -> Switch1/3
  Constant4/1 -> Switch1/1
  Switch1/1 -> CrCtl_st_mp/1
  CrCtl_stSub/1 -> Switch/3

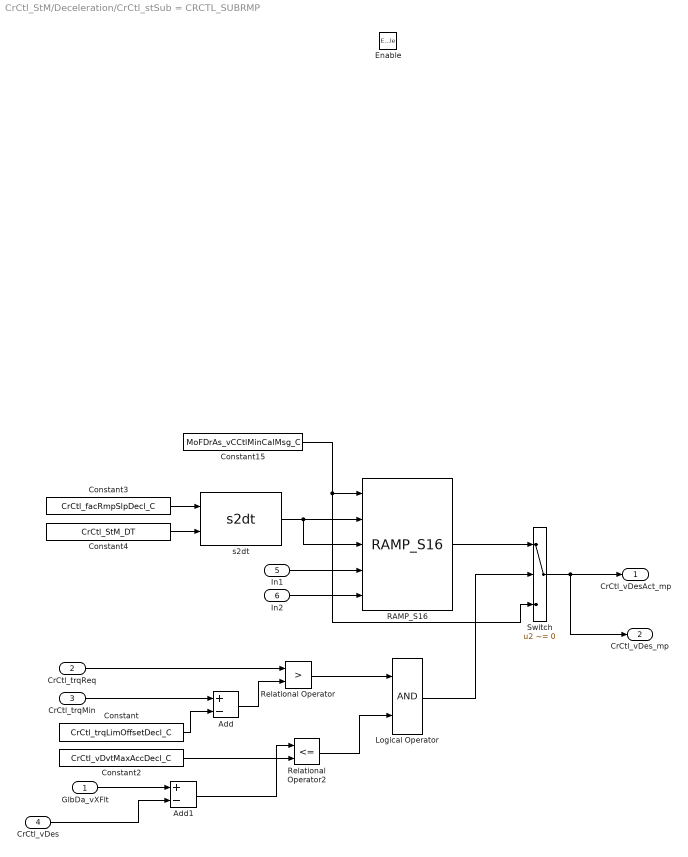
== system CrCtl_StM/Deceleration/CrCtl_stSub = CRCTL_SUBRMP ==
  GlbDa_vXFlt : Inport
  CrCtl_trqReq : Inport  Port=2
  CrCtl_trqMin : Inport  Port=3
  CrCtl_vDes : Inport  Port=4
  In1 : Inport  Port=5
  In2 : Inport  Port=6
  Enable : EnablePort
  Add : Sum  Inputs=+-
  Add1 : Sum  Inputs=+-
  Constant : Constant  Value=CrCtl_trqLimOffsetDecl_C
  Constant15 : Constant  Value=MoFDrAs_vCCtlMinCalMsg_C
  Constant2 : Constant  Value=CrCtl_vDvtMaxAccDecl_C
  Constant3 : Constant  Value=CrCtl_facRmpSlpDecl_C
  Constant4 : Constant  Value=CrCtl_StM_DT
  Logical Operator : Logic  AllPortsSameDT=off  OutDataTypeStr=boolean
  RAMP_S16 : CXLib/RAMP_S16
  Relational Operator : RelationalOperator  Operator=>  OutDataTypeStr=boolean  RndMeth=Simplest
  Relational Operator2 : RelationalOperator  Operator=<=  OutDataTypeStr=boolean  RndMeth=Simplest
  Switch : Switch  Criteria=u2 ~= 0
  s2dt : CXLib/s2dt
  CrCtl_vDesAct_mp : Outport
  CrCtl_vDes_mp : Outport  Port=2
  wires:
  CrCtl_trqReq/1 -> Relational Operator/1
  CrCtl_trqMin/1 -> Add/1
  Constant/1 -> Add/2
  Add/1 -> Relational Operator/2
  Relational Operator/1 -> Logical Operator/1
  GlbDa_vXFlt/1 -> Add1/1
  Add1/1 -> Relational Operator2/1
  Constant2/1 -> Relational Operator2/2
  s2dt/1 -> RAMP_S16/3, RAMP_S16/2
  Constant3/1 -> s2dt/1
  Constant4/1 -> s2dt/2
  In2/1 -> RAMP_S16/5
  CrCtl_vDes/1 -> Add1/2
  Logical Operator/1 -> Switch/2
  Relational Operator2/1 -> Logical Operator/2
  Switch/1 -> CrCtl_vDesAct_mp/1, CrCtl_vDes_mp/1
  RAMP_S16/1 -> Switch/1
  In1/1 -> RAMP_S16/4
  Constant15/1 -> Switch/3, RAMP_S16/1

== system CrCtl_StM/Deceleration/CrCtl_stSub = CRCTL_SUBRMPEND ==
  GlbDa_aXFlt : Inport
  GlbDa_vXFlt : Inport  Port=2
  CrCtl_vMax : Inport  Port=3
  CrCtl_st : Inport  Port=4
  Enable : EnablePort
  Constant1 : Constant  Value=CrCtl_aDeclThres_C
  Constant2 : Constant  Value=CrCtl_stSub_conv.CRCTL_SUBSTRTVAL
  Constant7 : Constant  Value=CruiseCtl_State_conv.CrCtl_CRUISE
  Constant8 : Constant  Value=CrCtl_stSub_conv.CRCTL_SUBPRECRUISE
  Constant9 : Constant  Value=CruiseCtl_State_conv.CrCtl_RESUME_F_ABOVE
  Logical Operator : Logic  Operator=NOT  AllPortsSameDT=off  OutDataTypeStr=boolean
  Logical Operator1 : Logic  Operator=OR  AllPortsSameDT=off  OutDataTypeStr=boolean
  MinMax : MinMax  Inputs=2
  Relational Operator : RelationalOperator  Operator=<  OutDataTypeStr=boolean  RndMeth=Simplest
  Relational Operator1 : RelationalOperator  Operator=>  OutDataTypeStr=boolean  RndMeth=Simplest
  Switch2 : Switch  Criteria=u2 ~= 0
  Switch4 : Switch  Criteria=u2 ~= 0
  Switch5 : Switch  Criteria=u2 ~= 0
  CrCtl_vDes_mp : Outport
  CrCtl_stSub_mp : Outport  Port=2
  CrCtl_st_mp : Outport  Port=3
  CrCtl_vDesAct_mp : Outport  Port=4
  wires:
  GlbDa_vXFlt/1 -> Relational Operator1/1, MinMax/1
  CrCtl_vMax/1 -> Relational Operator1/2, MinMax/2
  Constant7/1 -> Switch2/3
  Constant2/1 -> Switch4/1
  Constant8/1 -> Switch4/3
  Constant9/1 -> Switch5/1
  Switch2/1 -> Switch5/3
  Switch4/1 -> CrCtl_stSub_mp/1
  Switch5/1 -> CrCtl_st_mp/1
  GlbDa_aXFlt/1 -> Relational Operator/1
  Constant1/1 -> Relational Operator/2
  Relational Operator/1 -> Switch2/2, Logical Operator/1
  Relational Operator1/1 -> Switch5/2, Logical Operator1/1
  Logical Operator/1 -> Logical Operator1/2
  Logical Operator1/1 -> Switch4/2
  MinMax/1 -> CrCtl_vDesAct_mp/1, CrCtl_vDes_mp/1
  CrCtl_st/1 -> Switch2/1

== system CrCtl_StM/Deceleration/CrCtl_stSub = CRCTL_SUBSETEND ==
  GlbDa_vXFlt : Inport
  CrCtl_vMax : Inport  Port=2
  Enable : EnablePort
  Constant1 : Constant  Value=CruiseCtl_State_conv.CrCtl_CRUISE
  Constant3 : Constant  Value=CrCtl_stSub_conv.CRCTL_SUBSTRTVAL
  MinMax : MinMax  Inputs=2
  CrCtl_stSub_mp : Outport
  CrCtl_st_mp : Outport  Port=2
  CrCtl_vDes_mp : Outport  Port=3
  wires:
  Constant1/1 -> CrCtl_st_mp/1
  Constant3/1 -> CrCtl_stSub_mp/1
  GlbDa_vXFlt/1 -> MinMax/1
  CrCtl_vMax/1 -> MinMax/2
  MinMax/1 -> CrCtl_vDes_mp/1

== system CrCtl_StM/Deceleration/CrCtl_stSub = CRCTL_SUBSTRTVAL  ==
  GlbDa_vXFlt : Inport
  CrCtl_vMax : Inport  Port=2
  Enable : EnablePort
  Constant2 : Constant  Value=CrCtl_stSub_conv.CRCTL_SUBRMP
  MinMax : MinMax  Inputs=2
  Out2 : Outport
  CrCtl_stSub_mp : Outport  Port=2
  wires:
  GlbDa_vXFlt/1 -> MinMax/1
  CrCtl_vMax/1 -> MinMax/2
  MinMax/1 -> Out2/1
  Constant2/1 -> CrCtl_stSub_mp/1

== system CrCtl_StM/Off/CrCtl_stSub = CRCTL_SUBRMP ==
  CrCtl_trqReq : Inport
  PT_trqWhlMinEng : Inport  Port=2
  Enable : EnablePort
  Constant1 : Constant  Value=CrCtl_stSub_conv.CRCTL_SUBRMP
  Constant2 : Constant  Value=CruiseCtl_State_conv.CrCtl_OFF
  Constant3 : Constant  Value=CrCtl_stSub_conv.CRCTL_SUBNOSUB
  Constant5 : Constant  Value=CruiseCtl_State_conv.CrCtl_STAND_BY
  Relational Operator : RelationalOperator  Operator===  OutDataTypeStr=boolean  RndMeth=Simplest
  Switch : Switch  Criteria=u2 ~= 0
  Switch1 : Switch  Criteria=u2 ~= 0
  CrCtl_stSub_mp : Outport
  CrCtl_st_mp : Outport  Port=2
  wires:
  CrCtl_trqReq/1 -> Relational Operator/1
  PT_trqWhlMinEng/1 -> Relational Operator/2
  Relational Operator/1 -> Switch1/2, Switch/2
  Constant5/1 -> Switch1/1
  Constant3/1 -> Switch/1
  Constant1/1 -> Switch/3
  Constant2/1 -> Switch1/3
  Switch1/1 -> CrCtl_st_mp/1
  Switch/1 -> CrCtl_stSub_mp/1
